simulink subsystem "baro_filters"  (R2024b)
settings: Solver=VariableStepAuto  StartTime=0.0  StopTime=10.0  RelTol=1e-3
undefined symbols (not defined in the file or in its folder): airdata, dspblkCoreblockFVToolHelper, gcbh, GROUND_LEVEL, input_rate, pos_den, pos_num, position_init, use_custom_atm, vel_avg, vel_den, vel_num, velocity_init
libraries: simulink x1
settings Model: Creator=yevge  LastModifiedBy=Aiden Gaydos

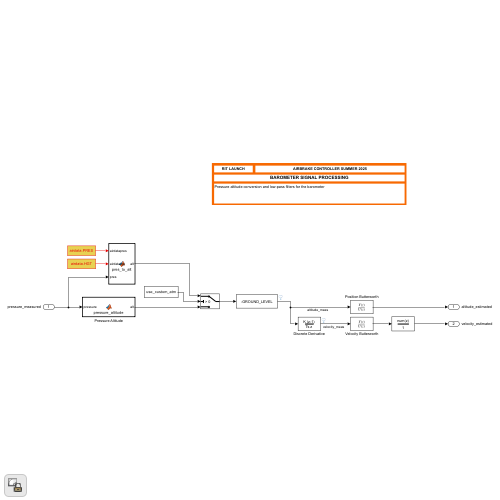
[thumbnail: Simulink's stored preview of the top-level diagram]
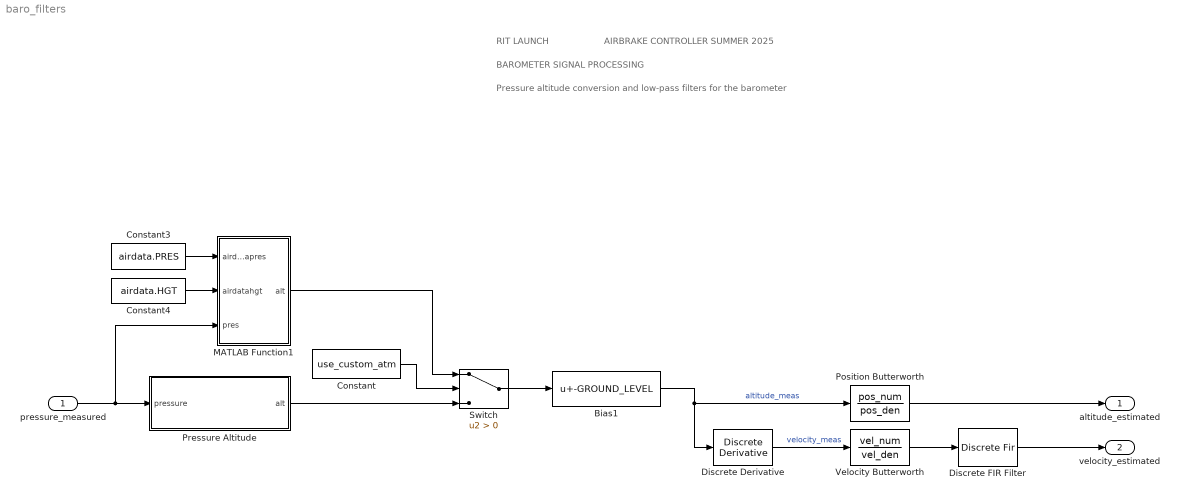
== system baro_filters ==
  note: BAROMETER SIGNAL PROCESSING
  note: Pressure altitude conversion and low-pass filters for the barometer
  note: RIT LAUNCH
  note: AIRBRAKE CONTROLLER SUMMER 2025
  pressure_measured : Inport  Unit=Pa  PortDimensions=1  SampleTime=1/input_rate
  Bias1 : Bias  Bias=-GROUND_LEVEL  SaturateOnIntegerOverflow=off
  Constant : Constant  Value=use_custom_atm
  Constant3 : Constant  Value=airdata.PRES
  Constant4 : Constant  Value=airdata.HGT
  Discrete Derivative : simulink/Discrete/Discrete Derivative  gainval=1.0  ICPrevScaledInput=0.0  OutMin=[]  OutMax=[]  OutDataType=fixdt(1, 16)  OutScaling=2^-10  DoSatur=off
  Discrete FIR Filter : DiscreteFir  LoadFcn=dspblkCoreblockFVToolHelper(gcbh,'load');  Coefficients=ones(1,vel_avg)/vel_avg
      settings: CopyFcn=dspblkCoreblockFVToolHelper(gcbh,'copy');  DeleteFcn=dspblkCoreblockFVToolHelper(gcbh,'close');  ModelCloseFcn=dspblkCoreblockFVToolHelper(gcbh,'close');  PreSaveFcn=dspblkCoreblockFVToolHelper(gcbh,'presave');  PostSaveFcn=dspblkCoreblockFVToolHelper(gcbh,'postsave');  CloseFcn=dspblkCoreblockFVToolHelper(gcbh,'close');
  MATLAB Function1 : MATLAB Function  TreatAsAtomicUnit=on
  Position Butterworth : DiscreteTransferFcn  LoadFcn=dspblkCoreblockFVToolHelper(gcbh,'load');  Numerator=pos_num  Denominator=pos_den  InitialStates=position_init(2)
      settings: CopyFcn=dspblkCoreblockFVToolHelper(gcbh,'copy');  DeleteFcn=dspblkCoreblockFVToolHelper(gcbh,'close');  ModelCloseFcn=dspblkCoreblockFVToolHelper(gcbh,'close');  PreSaveFcn=dspblkCoreblockFVToolHelper(gcbh,'presave');  PostSaveFcn=dspblkCoreblockFVToolHelper(gcbh,'postsave');  CloseFcn=dspblkCoreblockFVToolHelper(gcbh,'close');
  Pressure Altitude : MATLAB Function  TreatAsAtomicUnit=on
  Switch : Switch  Criteria=u2 > Threshold  SaturateOnIntegerOverflow=off  InputSameDT=off
  Velocity Butterworth : DiscreteTransferFcn  LoadFcn=dspblkCoreblockFVToolHelper(gcbh,'load');  Numerator=vel_num  Denominator=vel_den  InitialStates=velocity_init(2)
      settings: CopyFcn=dspblkCoreblockFVToolHelper(gcbh,'copy');  DeleteFcn=dspblkCoreblockFVToolHelper(gcbh,'close');  ModelCloseFcn=dspblkCoreblockFVToolHelper(gcbh,'close');  PreSaveFcn=dspblkCoreblockFVToolHelper(gcbh,'presave');  PostSaveFcn=dspblkCoreblockFVToolHelper(gcbh,'postsave');  CloseFcn=dspblkCoreblockFVToolHelper(gcbh,'close');
  altitude_estimated : Outport  Unit=m  PortDimensions=1
  velocity_estimated : Outport  Port=2  Unit=m/s  PortDimensions=1
  wires:
  Discrete Derivative/1 -> Velocity Butterworth/1  "velocity_meas"
  pressure_measured/1 -> Pressure Altitude/1(pressure), MATLAB Function1/3(pres)
  Bias1/1 -> Discrete Derivative/1, Position Butterworth/1  "altitude_meas"
  Position Butterworth/1 -> altitude_estimated/1
  Discrete FIR Filter/1 -> velocity_estimated/1
  Velocity Butterworth/1 -> Discrete FIR Filter/1
  Constant4/1 -> MATLAB Function1/2(airdatahgt)
  Constant3/1 -> MATLAB Function1/1(airdatapres)
  Switch/1 -> Bias1/1
  Pressure Altitude/1(alt) -> Switch/3
  Constant/1 -> Switch/2
  MATLAB Function1/1(alt) -> Switch/1

== matlab function baro_filters/Pressure Altitude ==
  data: pressure input; alt output
function alt = pressure_altitude(pressure)
    alt = (1 - (pressure ./ 101325).^(0.190284)) .* 145366.45 * 0.3048;
end

== matlab function baro_filters/MATLAB Function1 ==
  data: airdatapres input; airdatahgt input; pres input; alt output
function alt = pres_to_alt(airdatapres,airdatahgt,pres)
    alt = double(interp1(airdatapres,airdatahgt,pres,"linear","extrap"));
end
